simulink model "VibrationControl"  (R2020b)
settings: Solver=VariableStepAuto  StartTime=0.0  StopTime=10.0  RelTol=1e-3
undefined symbols (not defined in the file): DiscIntNeverNeededParam
libraries: pid_lib x1
settings Model: Creator=orangejuzi  LastModifiedBy=orangejuzi

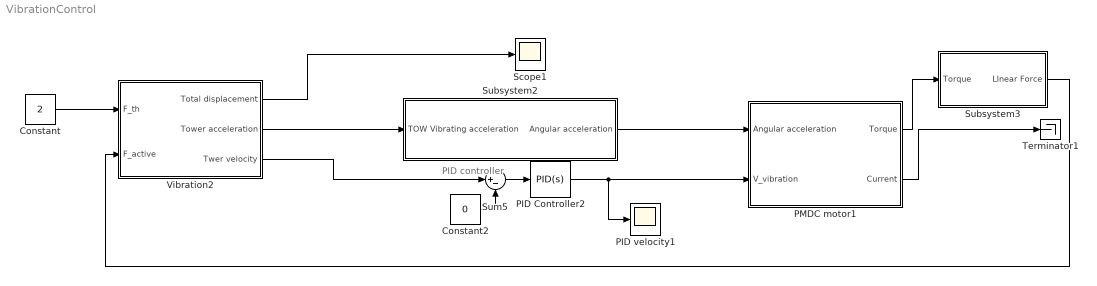
== system VibrationControl ==
  note: PID controller
  Constant : Constant  Value=2
  Constant2 : Constant  Value=0
  PID Controller2 : pid_lib/PID Controller  Controller=PID  Form=Parallel  TimeDomain=Continuous-time  UseExternalTs=off  SampleTime=-1  IntegratorMethod=Forward Euler  FilterMethod=Forward Euler  ControllerParametersSource=internal  P=-2000  I=-1  D=-1  UseFilter=on  N=597.035100888721  TunerSelectOption=Transfer Function Based (PID Tuner App)  InitialConditionSource=internal  InitialConditionForIntegrator=0  InitialConditionForFilter=0  DifferentiatorICPrevScaledInput=0  ExternalReset=none  TrackingMode=off  Kt=1  LimitOutput=off  SatLimitsSource=internal  UpperSaturationLimit=inf  LowerSaturationLimit=-inf  LinearizeAsGain=on  AntiWindupMode=none  Kb=1  POutMin=[]  POutMax=[]  IOutMin=[]  IOutMax=[]  DOutMin=[]  DOutMax=[]  NOutMin=[]  NOutMax=[]  SumOutMin=[]  SumOutMax=[]  SaturationOutMin=[]  SaturationOutMax=[]  PParamMin=[]  PParamMax=[]  IParamMin=[]  IParamMax=[]  DParamMin=[]  DParamMax=[]  NParamMin=[]  NParamMax=[]  KbParamMin=[]  KbParamMax=[]  KtParamMin=[]  KtParamMax=[]  KbOutMin=[]  KbOutMax=[]  KtOutMin=[]  KtOutMax=[]  IntegratorOutMin=[]  IntegratorOutMax=[]  FilterOutMin=[]  FilterOutMax=[]  SumI1OutMin=[]  SumI1OutMax=[]  SumI2OutMin=[]  SumI2OutMax=[]  SumI3OutMin=[]  SumI3OutMax=[]  SumI4OutMin=[]  SumI4OutMax=[]  SumDOutMin=[]  SumDOutMax=[]  DifferentiatorOutMin=[]  DifferentiatorOutMax=[]  FilterDiffOutCoefMin=[]  FilterDiffOutCoefMax=[]  ReciprocalOutMin=[]  ReciprocalOutMax=[]  SumDenOutMin=[]  SumDenOutMax=[]  SumNumOutMin=[]  SumNumOutMax=[]  DivideOutMin=[]  DivideOutMax=[]  UdiffTsProdOutMin=[]  UdiffTsProdOutMax=[]  NTsProdOutMin=[]  NTsProdOutMax=[]  UintegralTsProdOutMin=[]  UintegralTsProdOutMax=[]  UngainTsProdOutMin=[]  UngainTsProdOutMax=[]  IntegratorContinuousStateAttributes=''  IntegratorStateMustResolveToSignalObject=off  IntegratorRTWStateStorageClass=Auto  FilterContinuousStateAttributes=''  FilterStateMustResolveToSignalObject=off  FilterRTWStateStorageClass=Auto  ParallelPVariant=InternalParameters  IdealPVariant=Disabled  IVariant=InternalParameters  DVariant=InternalParameters  IntegratorVariant=Continuous  SatVariant=Disabled  AWVariant=Passthrough  PCopyVariant=Disabled  TRVariant=Disabled  FdbkBlocksVariant=Forward  IdealPFdbkVariant=Disabled  SatFdbkVariant=Disabled  DerivativeFilterVariant=ContFilter  NVariant=InternalParameters  NCopyVariant=Disabled  FilterICVariant=InternalICsFilter  IntegratorICVariant=InternalICs  ExternalResetVariant=Disabled  TRSumVariant=Passthrough  SumFdbkVariant=Disabled  SumVariant=Sum_PID  TsampFilterVariant=InternalTs  TsampNgainVariant=Passthrough  TsampIntegralVariant=Passthrough  ExternalSaturationOutDataTypeStr=Inherit: Same as second input
  PID velocity1 : Scope
  PMDC motor1 : Subsystem
  Scope1 : Scope
  Subsystem2 : Subsystem
  Subsystem3 : Subsystem
  Sum5 : Sum  Inputs=|+-
  Terminator1 : Terminator
  Vibration2 : Subsystem
  wires:
  Vibration2/2(Tower acceleration) -> Subsystem2/1(TOW Vibrating acceleration)
  Vibration2/3(Twer velocity) -> Sum5/1
  PID Controller2/1 -> PMDC motor1/2(V_vibration), PID velocity1/1
  PMDC motor1/1(Torque) -> Subsystem3/1(Torque)
  Subsystem2/1(Angular acceleration) -> PMDC motor1/1(Angular acceleration)
  PMDC motor1/2(Current) -> Terminator1/1
  Vibration2/1(Total displacement) -> Scope1/1
  Constant2/1 -> Sum5/2
  Subsystem3/1(LInear Force) -> Vibration2/2(F_active)
  Sum5/1 -> PID Controller2/1
  Constant/1 -> Vibration2/1(F_th)

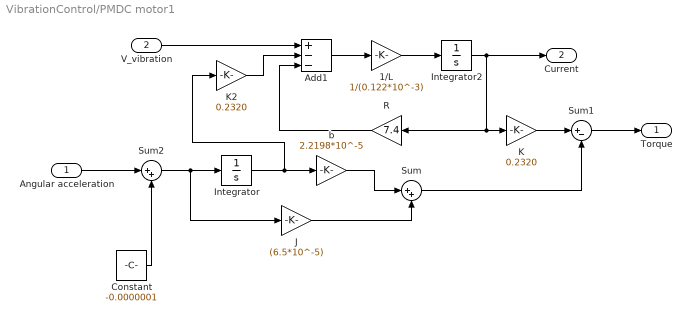
== system VibrationControl/PMDC motor1 ==
  Angular acceleration : Inport
  V_vibration : Inport  Port=2
  1/L : Gain  Gain=1/(0.122*10^-3)
  Add1 : Sum  Inputs=+--
  Constant : Constant  Value=-0.0000001
  Integrator : Integrator
  Integrator2 : Integrator
  J : Gain  Gain=(6.5*10^-5)
  K : Gain  Gain=0.2320
  K2 : Gain  Gain=0.2320
  R : Gain  Gain=7.4
  Sum : Sum  Inputs=|++
  Sum1 : Sum  Inputs=|+-
  Sum2 : Sum  Inputs=|++
  b : Gain  Gain=2.2198*10^-5
  Torque : Outport
  Current : Outport  Port=2
  wires:
  Sum1/1 -> Torque/1
  K2/1 -> Add1/2
  Integrator2/1 -> R/1, K/1, Current/1
  1/L/1 -> Integrator2/1
  Add1/1 -> 1/L/1
  K/1 -> Sum1/1
  R/1 -> Add1/3
  V_vibration/1 -> Add1/1
  Sum2/1 -> J/1, Integrator/1
  Integrator/1 -> K2/1, b/1
  b/1 -> Sum/1
  Sum/1 -> Sum1/2
  Constant/1 -> Sum2/2
  J/1 -> Sum/2
  Angular acceleration/1 -> Sum2/1

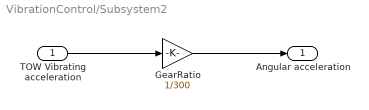
== system VibrationControl/Subsystem2 ==
  TOW Vibrating acceleration : Inport
  GearRatio : Gain  Gain=1/300
  Angular acceleration : Outport
  wires:
  TOW Vibrating acceleration/1 -> GearRatio/1
  GearRatio/1 -> Angular acceleration/1

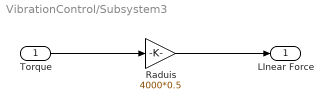
== system VibrationControl/Subsystem3 ==
  Torque : Inport
  Raduis : Gain  Gain=4000*0.5
  LInear Force : Outport
  wires:
  Torque/1 -> Raduis/1
  Raduis/1 -> LInear Force/1

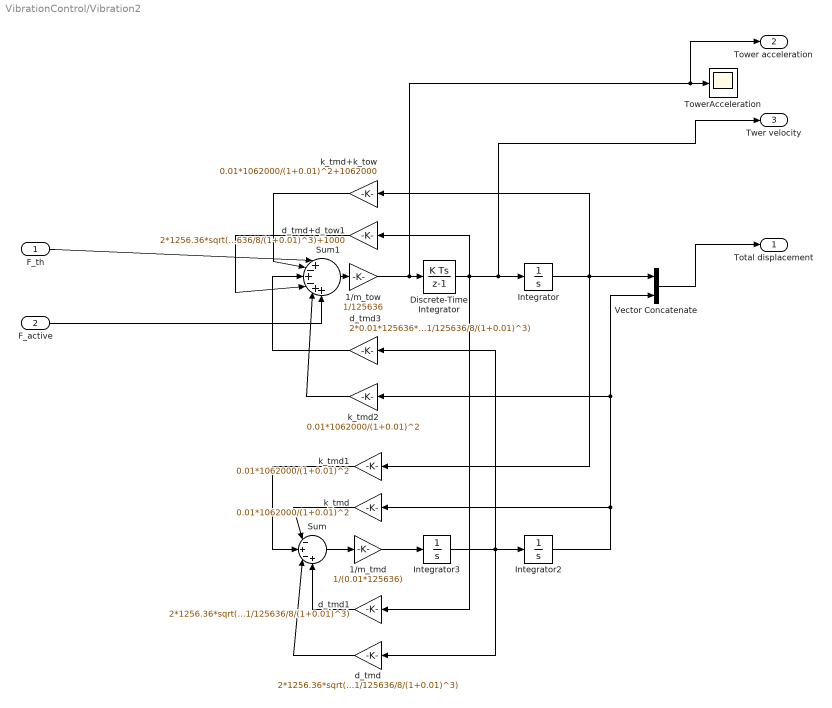
== system VibrationControl/Vibration2 ==
  F_th : Inport
  F_active : Inport  Port=2
  1/m_tmd : Gain  Gain=1/(0.01*125636)
  1/m_tow : Gain  Gain=1/125636
  Discrete-Time Integrator : DiscreteIntegrator  SampleTime=-1  ICPrevOutput=DiscIntNeverNeededParam  ICPrevScaledInput=DiscIntNeverNeededParam
  Integrator : Integrator
  Integrator2 : Integrator
  Integrator3 : Integrator
  Sum : Sum  Inputs=|-+-+
  Sum1 : Sum  Inputs=|+-+-++
  TowerAcceleration : Scope
  Vector Concatenate : Concatenate
  d_tmd : Gain  Gain=2*1256.36*sqrt(1062000/125636)*sqrt(1062000*3*0.01/125636/8/(1+0.01)^3)
  d_tmd+d_tow1 : Gain  Gain=2*1256.36*sqrt(1062000/125636)*sqrt(1062000*3*0.01/125636/8/(1+0.01)^3)+1000
  d_tmd1 : Gain  Gain=2*1256.36*sqrt(1062000/125636)*sqrt(1062000*3*0.01/125636/8/(1+0.01)^3)
  d_tmd3 : Gain  Gain=2*0.01*125636*sqrt(1062000*3*0.01/125636/8/(1+0.01)^3)
  k_tmd : Gain  Gain=0.01*1062000/(1+0.01)^2
  k_tmd+k_tow : Gain  Gain=0.01*1062000/(1+0.01)^2+1062000
  k_tmd1 : Gain  Gain=0.01*1062000/(1+0.01)^2
  k_tmd2 : Gain  Gain=0.01*1062000/(1+0.01)^2
  Total displacement : Outport
  Tower acceleration : Outport  Port=2
  Twer velocity : Outport  Port=3
  wires:
  Integrator/1 -> k_tmd+k_tow/1, Vector Concatenate/1, k_tmd1/1
  Integrator3/1 -> d_tmd/1, d_tmd3/1, Integrator2/1
  1/m_tmd/1 -> Integrator3/1
  Sum/1 -> 1/m_tmd/1
  1/m_tow/1 -> Discrete-Time Integrator/1, Tower acceleration/1, TowerAcceleration/1
  Sum1/1 -> 1/m_tow/1
  k_tmd/1 -> Sum/1
  d_tmd/1 -> Sum/3
  d_tmd1/1 -> Sum/4
  k_tmd1/1 -> Sum/2
  k_tmd+k_tow/1 -> Sum1/2
  d_tmd+d_tow1/1 -> Sum1/4
  d_tmd3/1 -> Sum1/3
  Integrator2/1 -> k_tmd/1, k_tmd2/1, Vector Concatenate/2
  k_tmd2/1 -> Sum1/5
  Vector Concatenate/1 -> Total displacement/1
  F_th/1 -> Sum1/1
  F_active/1 -> Sum1/6
  Discrete-Time Integrator/1 -> d_tmd+d_tow1/1, d_tmd1/1, Twer velocity/1, Integrator/1
